simulink model "simulink_entrega2_v2"  (R2024a)
settings: Solver=FixedStepAuto  StartTime=0.0  StopTime=500  FixedStep=Ts/10  RelTol=1e-3
undefined symbols (not defined in the file): K, q0, q1, q2, r0, r1, s0, s1, t0, tau, Ts
libraries: simulink x3

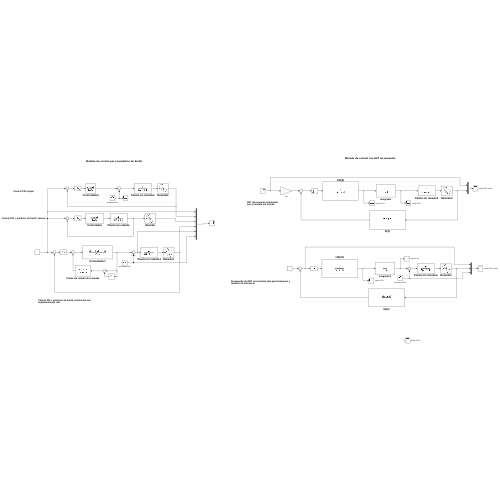
[thumbnail: Simulink's stored preview of the top-level diagram]
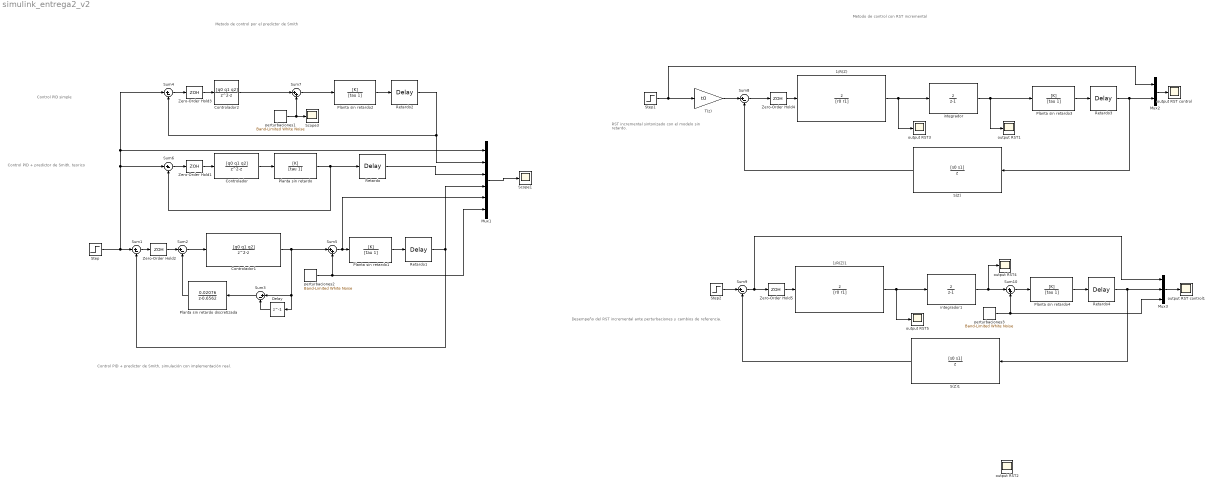
== system simulink_entrega2_v2 ==
  note: Control PID simple
  note: Metodo de control por el predictor de Smith
  note: Metodo de control con RST incremental
  note: Control PID + predictor de Smith, teorico
  note: Control PID + predictor de Smith, simulación con implementación real.
  note: RST incremental sintonizado
      | con el modelo sin retardo.
  note: Desempeño del RST incremental ante perturbaciones y cambios de referencia.
  1/R(Z) : DiscreteTransferFcn  Numerator=[1 0]  Denominator=[r0 r1]
  1/R(Z)1 : DiscreteTransferFcn  Numerator=[1 0]  Denominator=[r0 r1]
  Controlador : DiscreteTransferFcn  Numerator=[q0 q1 q2]  Denominator=[1 -1 0]
  Controlador1 : DiscreteTransferFcn  Numerator=[q0 q1 q2]  Denominator=[1 -1 0]
  Controlador2 : DiscreteTransferFcn  Numerator=[q0 q1 q2]  Denominator=[1 -1 0]
  Delay : Delay  DelayLength=1
  Mux1 : Mux  Inputs=6
  Mux2 : Mux  Inputs=2
  Mux3 : Mux  Inputs=3
  Planta sin retardo{,1..4} (5 alike) : TransferFcn  Numerator=[K]  Denominator=[tau 1]
  Planta sin retardo discretizada : DiscreteTransferFcn  Numerator=[0.02076]  Denominator=[1 -0.6562]
  Retardo{,1..4} (5 alike) : TransportDelay  DelayTime=2.2
  S(Z) : DiscreteTransferFcn  Numerator=[s0 s1]  Denominator=[1 0]
  S(Z)1 : DiscreteTransferFcn  Numerator=[s0 s1]  Denominator=[1 0]
  Scope1 : Scope
  Scope3 : Scope
  Step : Step  SampleTime=0
  Step1 : Step  SampleTime=0
  Step2 : Step  SampleTime=0
  Sum{1..4,6,8..9} (7 alike) : Sum  Inputs=|+-
  Sum10 : Sum  Inputs=|++
  Sum5 : Sum  Inputs=|++
  Sum7 : Sum  Inputs=|++
  T(z) : Gain  Gain=t0
  Zero-Order Hold{1..5} (5 alike) : ZeroOrderHold  SampleTime=Ts
  integrador : DiscreteTransferFcn  Numerator=[1 0]  Denominator=[1 -1]
  integrador1 : DiscreteTransferFcn  Numerator=[1 0]  Denominator=[1 -1]
  output RST control : Scope
  output RST control1 : Scope
  output RST{1..5} (5 alike) : Scope
  perturbaciones1 : simulink/Sources/Band-Limited White Noise  Cov=[300]  Ts=10*Ts  seed=[50892]  VectorParams1D=off
  perturbaciones2 : simulink/Sources/Band-Limited White Noise  Cov=[300]  Ts=10*Ts  seed=[50892]  VectorParams1D=off
  perturbaciones3 : simulink/Sources/Band-Limited White Noise  Cov=[300]  Ts=10*Ts  seed=[50892]  VectorParams1D=off
  wires:
  Planta sin retardo/1 -> Retardo/1, Sum6/2
  Mux1/1 -> Scope1/1
  Sum6/1 -> Zero-Order Hold1/1
  Controlador/1 -> Planta sin retardo/1
  Zero-Order Hold1/1 -> Controlador/1
  Controlador1/1 -> Sum5/1, Sum3/1, Delay/1
  Sum2/1 -> Controlador1/1
  Planta sin retardo1/1 -> Retardo1/1
  Retardo1/1 -> Mux1/4, Sum1/2
  Sum1/1 -> Zero-Order Hold2/1
  Planta sin retardo discretizada/1 -> Sum2/2
  Delay/1 -> Sum3/2
  Sum3/1 -> Planta sin retardo discretizada/1
  Zero-Order Hold2/1 -> Sum2/1
  Step/1 -> Sum6/1, Sum4/1, Mux1/1, Sum1/1
  Planta sin retardo2/1 -> Retardo2/1
  Sum4/1 -> Zero-Order Hold3/1
  Retardo2/1 -> Mux1/2, Sum4/2
  Zero-Order Hold3/1 -> Controlador2/1
  Sum5/1 -> Planta sin retardo1/1, Mux1/5
  perturbaciones1/1 -> Sum7/2, Scope3/1
  Sum7/1 -> Planta sin retardo2/1
  Controlador2/1 -> Sum7/1
  Mux2/1 -> output RST control/1
  Retardo3/1 -> S(Z)/1, Mux2/2
  Planta sin retardo3/1 -> Retardo3/1
  S(Z)/1 -> Sum8/2
  Step1/1 -> T(z)/1, Mux2/1
  T(z)/1 -> Sum8/1
  Zero-Order Hold4/1 -> 1/R(Z)/1
  Sum8/1 -> Zero-Order Hold4/1
  integrador/1 -> output RST1/1, Planta sin retardo3/1
  1/R(Z)/1 -> output RST3/1, integrador/1
  Retardo/1 -> Mux1/3
  perturbaciones2/1 -> Sum5/2, Mux1/6
  Planta sin retardo4/1 -> Retardo4/1
  S(Z)1/1 -> Sum9/2
  integrador1/1 -> Sum10/1, output RST4/1
  Sum9/1 -> Mux3/1, Zero-Order Hold5/1
  Zero-Order Hold5/1 -> 1/R(Z)1/1
  Step2/1 -> Sum9/1
  Retardo4/1 -> Mux3/2, S(Z)1/1
  1/R(Z)1/1 -> output RST5/1, integrador1/1
  Sum10/1 -> Planta sin retardo4/1
  perturbaciones3/1 -> Mux3/3, Sum10/2
  Mux3/1 -> output RST control1/1
